simulink model "l2"  (R2013a)
settings: Solver=ode45  StartTime=0.0  StopTime=30  RelTol=1e-3
settings Model: Creator=Sion  LastModifiedBy=Sion

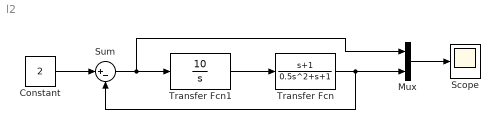
== system l2 ==
  Constant : Constant  Value=2
  Mux : Mux  Inputs=2
  Scope : Scope
      settings: TimeRange=30  YMin=-2.41672e-62  YMax=10  SaveName=ScopeData22
  Sum : Sum  Inputs=|+-
  Transfer Fcn : TransferFcn  Numerator=[1 1]  Denominator=[0.5 1 1]
  Transfer Fcn1 : TransferFcn  Numerator=[10]  Denominator=[1 0]
  wires:
  Transfer Fcn1/1 -> Transfer Fcn/1
  Transfer Fcn/1 -> Mux/2, Sum/2
  Constant/1 -> Sum/1
  Sum/1 -> Mux/1, Transfer Fcn1/1
  Mux/1 -> Scope/1
